simulink model "noisyStep"  (R2020b)
settings: Solver=VariableStepAuto  StartTime=0.0  StopTime=15  RelTol=1e-3
libraries: simulink x1
settings Model: Creator=Austin  LastModifiedBy=Austin

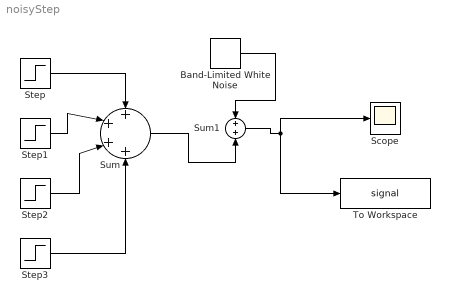
== system noisyStep ==
  Band-Limited White Noise : simulink/Sources/Band-Limited White Noise  Cov=[0.25]  Ts=0.1  seed=[23341]
  Scope : Scope
  Step : Step  Time=3  After=30  SampleTime=0
  Step1 : Step  Time=6  After=60  SampleTime=0
  Step2 : Step  Time=9  After=-45  SampleTime=0
  Step3 : Step  Time=11  After=60  SampleTime=0
  Sum : Sum  Inputs=++++
  Sum1 : Sum
  To Workspace : ToWorkspace  VariableName=signal  SampleTime=-1
  wires:
  Step/1 -> Sum/1
  Step2/1 -> Sum/3
  Band-Limited White Noise/1 -> Sum1/1
  Sum/1 -> Sum1/2
  Sum1/1 -> Scope/1, To Workspace/1
  Step1/1 -> Sum/2
  Step3/1 -> Sum/4
